simulink model "combinacion"  (Simulink 7.5)
settings: Solver=ode45  StartTime=0.0  StopTime=100.0  RelTol=1e-3
libraries: fuzblock x1, simulink_need_slupdate x1
settings Model: Creator=manu  LastModifiedBy=manu

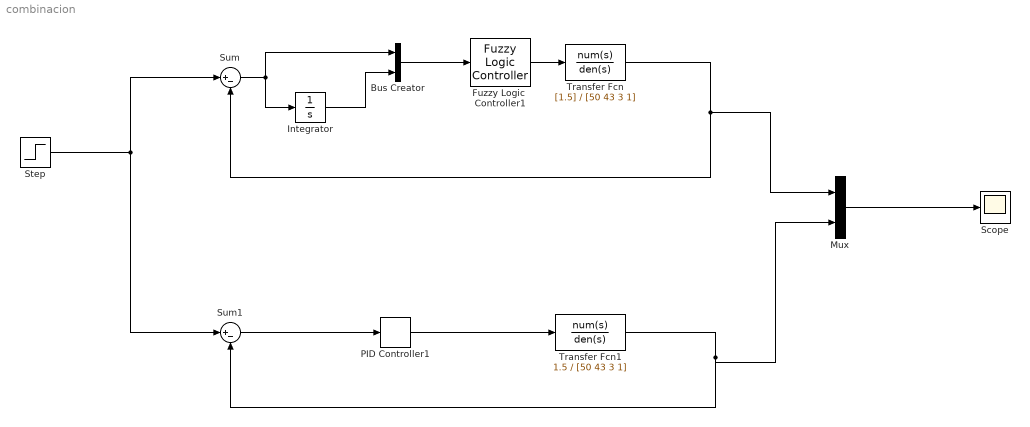
== system combinacion ==
  Bus Creator : BusCreator  Inputs=2
  Fuzzy Logic  Controller1 : fuzblock/Fuzzy Logic  Controller  SystemSampleTime=-1  fis='sistema_mamdani.fis'
  Integrator : Integrator
  Mux : Mux  Inputs=2
  PID Controller1 : simulink_need_slupdate/PID Controller  SystemSampleTime=-1  P=6.36  I=0.4968  D=20.3561
  Scope : Scope
      settings: TimeRange=100  YMin=0  YMax=1.4
  Step : Step  SampleTime=0
  Sum : Sum  Inputs=|+-
  Sum1 : Sum  Inputs=|+-  OutDataType=sfix(16)  OutScaling=2^0  SaturateOnIntegerOverflow=on  InputSameDT=on  OutDataTypeStr=Inherit: Same as first input
  Transfer Fcn : TransferFcn  Numerator=[1.5]  Denominator=[50 43 3 1]
  Transfer Fcn1 : TransferFcn  Numerator=1.5  Denominator=[50 43 3 1]
  wires:
  Fuzzy Logic  Controller1/1 -> Transfer Fcn/1
  Sum/1 -> Bus Creator/1, Integrator/1
  Bus Creator/1 -> Fuzzy Logic  Controller1/1
  Transfer Fcn/1 -> Sum/2, Mux/1
  Integrator/1 -> Bus Creator/2
  PID Controller1/1 -> Transfer Fcn1/1
  Sum1/1 -> PID Controller1/1
  Step/1 -> Sum1/1, Sum/1
  Transfer Fcn1/1 -> Sum1/2, Mux/2
  Mux/1 -> Scope/1
